simulink model "simulacion_simulink"  (R2016b)
settings: Solver=VariableStepAuto  StartTime=0.0  StopTime=10.0  RelTol=1e-3
settings Model: Creator=Mauricio  LastModifiedBy=Mauricio

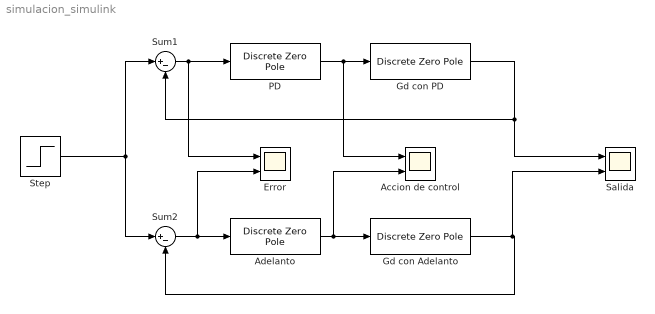
== system simulacion_simulink ==
  Accion de control : Scope  NumInputPorts=2
  Adelanto : DiscreteZeroPole  Zeros=[0.7723]  Poles=[0.724]  Gain=0.032954  SampleTime=0.15
  Error : Scope  NumInputPorts=2
  Gd con Adelanto : DiscreteZeroPole  Zeros=[0.1608]  Poles=[1 0.7408]  Gain=2.3164  SampleTime=0.15
  Gd con PD : DiscreteZeroPole  Zeros=[0.1608]  Poles=[1 0.7408]  Gain=2.3164  SampleTime=0.15
  PD : DiscreteZeroPole  Zeros=[0.455]  Poles=[0]  Gain=0.061627  SampleTime=0.15
  Salida : Scope  NumInputPorts=2
  Step : Step  Time=0  SampleTime=0.15
  Sum1 : Sum  Inputs=|+-
  Sum2 : Sum  Inputs=|+-
  wires:
  Sum1/1 -> Error/1, PD/1
  Gd con PD/1 -> Sum1/2, Salida/1
  PD/1 -> Accion de control/1, Gd con PD/1
  Step/1 -> Sum1/1, Sum2/1
  Sum2/1 -> Error/2, Adelanto/1
  Gd con Adelanto/1 -> Salida/2, Sum2/2
  Adelanto/1 -> Accion de control/2, Gd con Adelanto/1
